simulink model "Copy_of_minimal_rcu_full"  (R2014b)
settings: Solver=ode4  SolverMode=SingleTasking  StartTime=0.0  StopTime=t_sim  FixedStep=sample_time_model  RelTol=1e-3
PreLoadFcn:
  | initModell
InitFcn:
  | initModell
undefined symbols (not defined in the file): FILTER_TAU_EXT, FIXED_FILTER_BANDWIDTH, FIXED_FILTER_BANDWIDTH_OBSERVER, iter, K_INV, KI2TAU_VEC, KS_trq, KT_trq, load_inertia, load_mass, MAX_CURRENT, MIN_SING_VALUE_M_CART, q0, rCEE_i, sample_time_model, sample_time_robot, tau_max
libraries: simulink x69, robotics x15, beasty_sfcns x7, lwr_dynamics x6, trafo3dLib x4, holgersRobLib x3, dspmtrx3 x1, dspinverses x1
(part 3 of 4)

== system Copy_of_minimal_rcu_full/Roboter+controller/controller/Cartesian Impedance Control/Subsystem/Cartesian Compliance Control/Iterative Computation of the 'Stiffness' and Gravity Compensation ==
  note: Notice that q_bar is chosen after the delay block
      | while the tau_qbar is computed before the delay.
      | Therefore, the signals q_bar and tau_qbar fit together
      | and the last iteration step is used only to compute the
      | output not for an update of q_bar!
  q_m : Inport
  type : Inport  Port=2
  niter : Inport  Port=3
  Kd : Inport  Port=4
  Hsd : Inport  Port=5
  load : Inport  Port=6
  tcp_offset : Inport  Port=7
  base_acceleration : Inport  Port=8
  relaxing : Inport  Port=9
  For Iterator : ForIterator  ResetStates=reset  IterationSource=external  IterationLimit=iter+1  ShowIterationPort=off
  Iteration Step : Subsystem
  Iteration for Nolcos Controller : Subsystem
  Terminator : Terminator
  Unit Delay External IC : simulink/Additional Math & Discrete/Additional Discrete/Unit Delay External IC  tsamp=-1
  q_bar : Outport
  tau_qbar : Outport  Port=2
  Jx_bar : Outport  Port=3
  F : Outport  Port=4
  tau_stiffness : Outport  Port=5
  tau_grav : Outport  Port=6
  wires:
  Iteration for Nolcos Controller/3(grav) -> tau_grav/1
  Iteration for Nolcos Controller/6(tau_stiffness) -> tau_stiffness/1
  base_acceleration/1 -> Iteration for Nolcos Controller/7(base_acceleration)
  niter/1 -> For Iterator/1
  Iteration for Nolcos Controller/2(Jx(q)) -> Jx_bar/1
  load/1 -> Iteration for Nolcos Controller/3(load)
  Hsd/1 -> Iteration for Nolcos Controller/2(Hsd)
  Kd/1 -> Iteration for Nolcos Controller/4(Kd)
  Iteration for Nolcos Controller/1(l(q)) -> tau_qbar/1, Iteration Step/1(l(q))
  q_m/1 -> Iteration Step/2(theta), Unit Delay External IC/2
  Unit Delay External IC/1 -> q_bar/1, Iteration for Nolcos Controller/1(q)
  Iteration Step/1(q_bar) -> Unit Delay External IC/1
  type/1 -> Iteration for Nolcos Controller/5(type)
  Iteration for Nolcos Controller/5(F) -> F/1
  tcp_offset/1 -> Iteration for Nolcos Controller/6(tcp_offset)
  relaxing/1 -> Iteration for Nolcos Controller/8(relaxing)
  Iteration for Nolcos Controller/4(Fkin) -> Terminator/1

== system Copy_of_minimal_rcu_full/Roboter+controller/controller/Cartesian Impedance Control/Subsystem/Cartesian Compliance Control/Nullspace Stiffness1 ==
  P_inv : Inport
  0_JT_4 : Inport  Port=2
  dtheta : Inport  Port=3
  M : Inport  Port=4
  desiredVec : Inport  Port=5
  K : Inport  Port=6
  D : Inport  Port=7
  O_T_4 : Inport  Port=8
  W_T_O : Inport  Port=9
  Enable : EnablePort
  Product : Product  Multiplication=Matrix(*)  RndMeth=Zero
  Product2 : Product  Multiplication=Matrix(*)  RndMeth=Zero
  Product4 : Product  Multiplication=Matrix(*)  RndMeth=Zero
  Reshape : Reshape  OutputDimensionality=Column vector (2-D)
  Reshape1 : Reshape  OutputDimensions=[7,6]
  Reshape2 : Reshape  OutputDimensionality=Customize  OutputDimensions=[4,4]
  Reshape3 : Reshape  OutputDimensionality=Column vector (2-D)
  Reshape4 : Reshape
  Reshape5 : Reshape  OutputDimensionality=Customize  OutputDimensions=[7,6]
  Selector : Selector  NumberOfDimensions=2  InputPortWidth=3  IndexOptions=Index vector (dialog),Index vector (dialog)  Indices=[1 2 3],[1 2 3]  OutputSizes=1,1
  Stiffness Calculation : Subsystem
  Transpose : Math  Operator=transpose  SaturateOnIntegerOverflow=on
  tau : Outport  OutDataTypeStr=double  PortDimensions=7  OutputWhenDisabled=reset  InitialOutput=zeros(1,7)
  wires:
  Stiffness Calculation/1(0_F_stiff) -> Product4/2
  M/1 -> Stiffness Calculation/7(Mass)
  K/1 -> Stiffness Calculation/4(Stiffness)
  D/1 -> Stiffness Calculation/6(damping)
  O_T_4/1 -> Stiffness Calculation/2(0_T_4)
  dtheta/1 -> Stiffness Calculation/5(qd)
  Reshape1/1 -> Reshape3/1
  P_inv/1 -> Product2/1
  Product4/1 -> Reshape1/1
  Product2/1 -> Reshape4/1
  0_JT_4/1 -> Reshape5/1
  W_T_O/1 -> Reshape2/1
  Reshape2/1 -> Selector/1
  Product/1 -> Stiffness Calculation/3(Ellbow_Field)
  Selector/1 -> Transpose/1  "W_R_O"
  desiredVec/1 -> Reshape/1
  Transpose/1 -> Product/1  "O_R_W"
  Reshape/1 -> Product/2
  Reshape3/1 -> Product2/2
  Reshape4/1 -> tau/1
  Reshape5/1 -> Stiffness Calculation/1(O_JT_4), Product4/1

== system Copy_of_minimal_rcu_full/Roboter+controller/controller/Cartesian Impedance Control/Subsystem/Cartesian Compliance Control/Singularity Avoidance ==
  qm : Inport
  dqm : Inport  Port=2
  dist : Inport  Port=3
  gain : Inport  Port=4
  d_sing : Inport  Port=5
  Enable : EnablePort  StatesWhenEnabling=reset
  Add : Sum
  Gain : Gain  Gain=-1
  Product : Product  Multiplication=Matrix(*)  RndMeth=Zero
  Product1 : Product  RndMeth=Zero
  Proj. : MATLAB Function  TreatAsAtomicUnit=on
  Reshape : Reshape  OutputDimensionality=Column vector (2-D)
  Reshape1 : Reshape
  Singularity Avoidance : S-Function  FunctionName=lbr_singul_avoid_sfun  Parameters=robot  EnableBusSupport=off  mask{robot=KUKA-LBR}
      mask help: Singularity Avoidance Torques for the DLR lightweight robots
      mask TypeOptions robot: LBR-II | LBR-M | KUKA-LBR
      mask Display:
      | port_label('input', 1, 'q')
      | port_label('input', 2, 'distance')
      | port_label('input', 3, 'gain')
      | port_label('output', 1, 'tau')
      | port_label('output', 2, 'index')
  tau : Outport  OutDataTypeStr=double  PortDimensions=7  OutputWhenDisabled=reset  InitialOutput=zeros(1,7)
  index : Outport  Port=2  OutDataTypeStr=double  PortDimensions=1  OutputWhenDisabled=reset  InitialOutput=0
  wires:
  Singularity Avoidance/1 -> Proj./1(tau), Add/2
  qm/1 -> Singularity Avoidance/1
  dist/1 -> Singularity Avoidance/2
  gain/1 -> Singularity Avoidance/3
  Singularity Avoidance/2 -> index/1
  Proj./1(P) -> Product/1
  dqm/1 -> Reshape/1
  Product/1 -> Reshape1/1
  d_sing/1 -> Product1/1
  Product1/1 -> Gain/1
  Gain/1 -> Add/1
  Add/1 -> tau/1
  Reshape/1 -> Product/2
  Reshape1/1 -> Product1/2

== system Copy_of_minimal_rcu_full/Roboter+controller/controller/Cartesian Impedance Control/Subsystem/Cartesian Compliance Control/cmd ==
  all : Inport
  Embedded MATLAB Function1 : MATLAB Function  TreatAsAtomicUnit=on
  Select K_diag : Selector  InputPortWidth=23  Indices=[3:8]
  Select Type : Selector  InputPortWidth=23
  Select niter : Selector  InputPortWidth=23  Indices=2
  type : Outport
  niter : Outport  Port=2
  K_diag : Outport  Port=3
  wires:
  all/1 -> Select Type/1, Select niter/1, Select K_diag/1
  Select Type/1 -> type/1
  Select niter/1 -> niter/1
  Select K_diag/1 -> Embedded MATLAB Function1/1(K_diag)
  Embedded MATLAB Function1/1(K) -> K_diag/1

== system Copy_of_minimal_rcu_full/Roboter+controller/controller/Cartesian Impedance Control/Subsystem/Cartesian Compliance Control/cmd2 ==
  all : Inport
  Embedded MATLAB Function1 : MATLAB Function  TreatAsAtomicUnit=on
  Select K_diag : Selector  InputPortWidth=23  Indices=[3:8]
  Select Type : Selector  InputPortWidth=23  Indices=23
  Select niter : Selector  InputPortWidth=23  Indices=[9:14]
  xi_diag : Outport
  damping_type : Outport  Port=2
  K_diag : Outport  Port=3
  K_sqrt : Outport  Port=4
  wires:
  Select K_diag/1 -> Embedded MATLAB Function1/1(K_diag)
  Select Type/1 -> damping_type/1
  all/1 -> Select K_diag/1, Select niter/1, Select Type/1
  Embedded MATLAB Function1/1(K) -> K_diag/1
  Embedded MATLAB Function1/2(K_sqrt) -> K_sqrt/1
  Select niter/1 -> xi_diag/1

== system Copy_of_minimal_rcu_full/Roboter+controller/controller/Cartesian Impedance Control/Subsystem/Cartesian Compliance Control/cmd3 ==
  all : Inport
  Select K_diag : Selector  InputPortWidth=23  Indices=16
  Select Type : Selector  InputPortWidth=23  Indices=[17:19]
  Select niter : Selector  InputPortWidth=23  Indices=15
  desiredVec : Outport
  K_NS : Outport  Port=2
  Xi_NS : Outport  Port=3
  wires:
  all/1 -> Select Type/1, Select niter/1, Select K_diag/1
  Select Type/1 -> desiredVec/1
  Select niter/1 -> K_NS/1
  Select K_diag/1 -> Xi_NS/1

== system Copy_of_minimal_rcu_full/Roboter+controller/controller/Cartesian Impedance Control/Subsystem/Cartesian Compliance Control/cmd4 ==
  all : Inport
  Select K_diag : Selector  InputPortWidth=23  Indices=22
  Select Type : Selector  InputPortWidth=23  Indices=20
  Select niter : Selector  InputPortWidth=23  Indices=21
  sing_dist : Outport
  sing_gain : Outport  Port=2
  sing_damp : Outport  Port=3
  wires:
  Select K_diag/1 -> sing_damp/1
  Select niter/1 -> sing_gain/1
  Select Type/1 -> sing_dist/1
  all/1 -> Select K_diag/1, Select niter/1, Select Type/1

== system Copy_of_minimal_rcu_full/Roboter+controller/controller/Cartesian Impedance Control/calculate Feedforward/Numerische Differentiation/Rotate_wrench1 ==
  A_T_B : Inport
  0 : Constant  Value=zeros(3,3)  VectorParams1D=off
  Matrix Concatenation : Concatenate  Mode=Multidimensional array  ConcatenateDimension=2
  Matrix Concatenation1 : Concatenate  Mode=Multidimensional array
  Matrix Concatenation2 : Concatenate  Mode=Multidimensional array  ConcatenateDimension=2
  R : Selector  NumberOfDimensions=2  InputPortWidth=3  IndexOptions=Index vector (dialog),Index vector (dialog)  Indices=[1,2,3],[1 2 3]
  A_R_B : Outport
  wires:
  Matrix Concatenation1/1 -> A_R_B/1
  Matrix Concatenation2/1 -> Matrix Concatenation1/2
  Matrix Concatenation/1 -> Matrix Concatenation1/1
  0/1 -> Matrix Concatenation2/1, Matrix Concatenation/2
  A_T_B/1 -> R/1
  R/1 -> Matrix Concatenation/1, Matrix Concatenation2/2

== system Copy_of_minimal_rcu_full/Roboter+controller/controller/Cartesian Impedance Control/calculate Feedforward/Numerische Differentiation/nan_chk4 ==
  in : Inport
  Add : Sum
  Compare To Zero : simulink/Logic and Bit Operations/Compare To Zero  relop===  OutDataTypeStr=uint8  ZeroCross=off
  Compare To Zero1 : simulink/Logic and Bit Operations/Compare To Zero  relop=>  OutDataTypeStr=uint8  ZeroCross=off
  Constant2 : Constant  Value=sample_time_model
  Discrete Derivative2 : simulink/Discrete/Discrete Derivative  gainval=1.0  ICPrevScaledInput=0.0  InputProcessing=Inherited  OutMin=[]  OutMax=[]  OutDataType=sfix(16)  OutScaling=2^-10  DoSatur=off
  NAN_chk_theta : Display
  Product1 : Product  RndMeth=Zero
  Relational Operator : RelationalOperator  Operator===  OutDataTypeStr=boolean
  Sum of Elements : Sum  Inputs=+
  Switch : Switch  Criteria=u2 > Threshold
  Unit Delay1 : UnitDelay  SampleTime=-1
  in_checked : Outport
  wires:
  Unit Delay1/1 -> Switch/1
  Add/1 -> Unit Delay1/1
  Product1/1 -> Add/2
  Discrete Derivative2/1 -> Product1/1
  Constant2/1 -> Product1/2
  Switch/1 -> Add/1, Discrete Derivative2/1, in_checked/1
  in/1 -> Switch/3, Relational Operator/2, Relational Operator/1
  Relational Operator/1 -> Compare To Zero/1
  Compare To Zero/1 -> Sum of Elements/1
  Sum of Elements/1 -> Compare To Zero1/1
  Compare To Zero1/1 -> Switch/2, NAN_chk_theta/1

== system Copy_of_minimal_rcu_full/Roboter+controller/controller/Cartesian Impedance Control/calculate Feedforward/Numerische Differentiation/numerical differentiation ==
  note: 0_dx = [0_dx_trans; 0_dx_rot]
  note: 0_dx_trans calcualated by numerical differentiation of the position of T_desired
  note: 0_dx_rot calculated by numerical differentiation
      | omegatilde = dR/dt*R^T
  T_des : Inport
  Derivative1 : Derivative
  Derivative2 : Derivative
  Math Function : Math  Operator=transpose  SaturateOnIntegerOverflow=on
  Mux : Mux
  Product3 : Product  Multiplication=Matrix(*)  RndMeth=Zero
  Reshape7 : Reshape  OutputDimensionality=Column vector (2-D)  OutputDimensions=[7,6]
  select_-omega_x : Selector  NumberOfDimensions=2  InputPortWidth=3  IndexOptions=Index vector (dialog),Index vector (dialog)  Indices=3,2  OutputSizes=1,1
  select_omega_y : Selector  NumberOfDimensions=2  InputPortWidth=3  IndexOptions=Index vector (dialog),Index vector (dialog)  Indices=1,3  OutputSizes=1,1
  select_omega_z : Selector  NumberOfDimensions=2  InputPortWidth=3  IndexOptions=Index vector (dialog),Index vector (dialog)  Indices=2,1  OutputSizes=1,1
  select_rot : Selector  NumberOfDimensions=2  InputPortWidth=3  IndexOptions=Index vector (dialog),Index vector (dialog)  Indices=[1:3],[1:3]  OutputSizes=1,1
  select_trans : Selector  NumberOfDimensions=2  InputPortWidth=3  IndexOptions=Index vector (dialog),Index vector (dialog)  Indices=[1:3],4  OutputSizes=1,1
  0_dx : Outport
  wires:
  select_rot/1 -> Derivative1/1, Math Function/1
  Derivative1/1 -> Product3/1
  Math Function/1 -> Product3/2
  select_trans/1 -> Derivative2/1
  Product3/1 -> select_-omega_x/1, select_omega_y/1, select_omega_z/1
  select_-omega_x/1 -> Mux/2
  select_omega_z/1 -> Mux/4
  select_omega_y/1 -> Mux/3
  Derivative2/1 -> Mux/1  "0_dx_trans"
  Mux/1 -> Reshape7/1
  T_des/1 -> select_rot/1, select_trans/1
  Reshape7/1 -> 0_dx/1

== system Copy_of_minimal_rcu_full/Roboter+controller/controller/Cartesian Impedance Control/easy interpolate/easy interpolator inside/correct sign ==
  In1 : Inport
  In2 : Inport  Port=2
  Constant2 : Constant
  Constant3 : Constant  Value=-1
  Relational Operator : RelationalOperator  Operator=<  OutDataTypeStr=boolean
  Switch : Switch  Criteria=u2 > Threshold
  Out1 : Outport
  wires:
  Switch/1 -> Out1/1
  In1/1 -> Relational Operator/1
  Constant2/1 -> Switch/1
  Relational Operator/1 -> Switch/2
  Constant3/1 -> Switch/3
  In2/1 -> Relational Operator/2

== system Copy_of_minimal_rcu_full/Roboter+controller/controller/Cartesian Impedance Control/easy interpolate/easy interpolator inside/memorize last ==
  In1 : Inport
  Detect Change : simulink/Logic and Bit Operations/Detect Change  vinit=0  InputProcessing=Inherited  OutDataTypeStr=uint8
  Display1 : Display
  Display2 : Display
  Display3 : Display
  Scope : Scope
      settings: YMin=1  YMax=1
  Triggered Subsystem : Subsystem  TreatAsAtomicUnit=on
  Unit Delay : UnitDelay  SampleTime=-1
  Out1 : Outport
  wires:
  In1/1 -> Display3/1, Detect Change/1, Unit Delay/1
  Detect Change/1 -> Triggered Subsystem/Trigger, Display1/1, Scope/1
  Unit Delay/1 -> Triggered Subsystem/1(In1)
  Triggered Subsystem/1(Out1) -> Out1/1, Display2/1

== system Copy_of_minimal_rcu_full/Roboter+controller/controller/Joint Impedance/JOINT_IMPEDANCE_CONTROL/Joint Compliance Control/Damping Design via Generalized Eigenvalues ==
  note: The following is satisfied:
      |   V'BV=I
      |   inv(V)*inv(B)*A*V=diag(lam)
      |   H=inv(V')=B*V-->B=H*H' and B=inv(V')*inv(V)
      |   The damping should thus be chosen as Dc = H*diag(d0)*H'
  M : Inport
  K : Inport  Port=2
  damp_fac : Inport  Port=3
  Damping Design via Generalized Eigenvalues QR right : Subsystem
  D : Outport
  wires:
  damp_fac/1 -> Damping Design via Generalized Eigenvalues QR right/3(damp_fac)
  K/1 -> Damping Design via Generalized Eigenvalues QR right/1(K)
  M/1 -> Damping Design via Generalized Eigenvalues QR right/2(M)
  Damping Design via Generalized Eigenvalues QR right/1(D) -> D/1

== system Copy_of_minimal_rcu_full/Roboter+controller/controller/Joint Impedance/JOINT_IMPEDANCE_CONTROL/Joint Compliance Control/NAN_checks ==
  D : Inport
  qm : Inport  Port=2
  dqm : Inport  Port=3
  qm_d : Inport  Port=4
  K_diag : Inport  Port=5
  stiffness correction : Inport  Port=6
  g(theta) : Inport  Port=7
  tau : Inport  Port=8
  NAN_chk_K_diag : Display
  NAN_chk_damping : Display
  NAN_chk_gravitation : Display
  NAN_chk_stiffness correction : Display
  NAN_chk_tau_joint_impedance : Display
  NAN_chk_theta_dot_measured : Display
  NAN_chk_theta_measured : Display
  NAN_chk_theta_measured_desired : Display
  hold_zero_if_nan_or_inf1 : Subsystem
  hold_zero_if_nan_or_inf2 : Subsystem
  hold_zero_if_nan_or_inf3 : Subsystem
  hold_zero_if_nan_or_inf4 : Subsystem
  hold_zero_if_nan_or_inf5 : Subsystem
  hold_zero_if_nan_or_inf6 : Subsystem
  hold_zero_if_nan_or_inf7 : Subsystem
  hold_zero_if_nan_or_inf8 : Subsystem
  wires:
  hold_zero_if_nan_or_inf2/1(Out1) -> NAN_chk_theta_measured/1
  hold_zero_if_nan_or_inf3/1(Out1) -> NAN_chk_theta_dot_measured/1
  hold_zero_if_nan_or_inf4/1(Out1) -> NAN_chk_theta_measured_desired/1
  hold_zero_if_nan_or_inf5/1(Out1) -> NAN_chk_K_diag/1
  hold_zero_if_nan_or_inf6/1(Out1) -> NAN_chk_damping/1
  hold_zero_if_nan_or_inf7/1(Out1) -> NAN_chk_stiffness correction/1
  hold_zero_if_nan_or_inf8/1(Out1) -> NAN_chk_gravitation/1
  qm/1 -> hold_zero_if_nan_or_inf2/1(In1)
  dqm/1 -> hold_zero_if_nan_or_inf3/1(In1)
  qm_d/1 -> hold_zero_if_nan_or_inf4/1(In1)
  K_diag/1 -> hold_zero_if_nan_or_inf5/1(In1)
  D/1 -> hold_zero_if_nan_or_inf6/1(In1)
  stiffness correction/1 -> hold_zero_if_nan_or_inf7/1(In1)
  g(theta)/1 -> hold_zero_if_nan_or_inf8/1(In1)
  hold_zero_if_nan_or_inf1/1(Out1) -> NAN_chk_tau_joint_impedance/1
  tau/1 -> hold_zero_if_nan_or_inf1/1(In1)

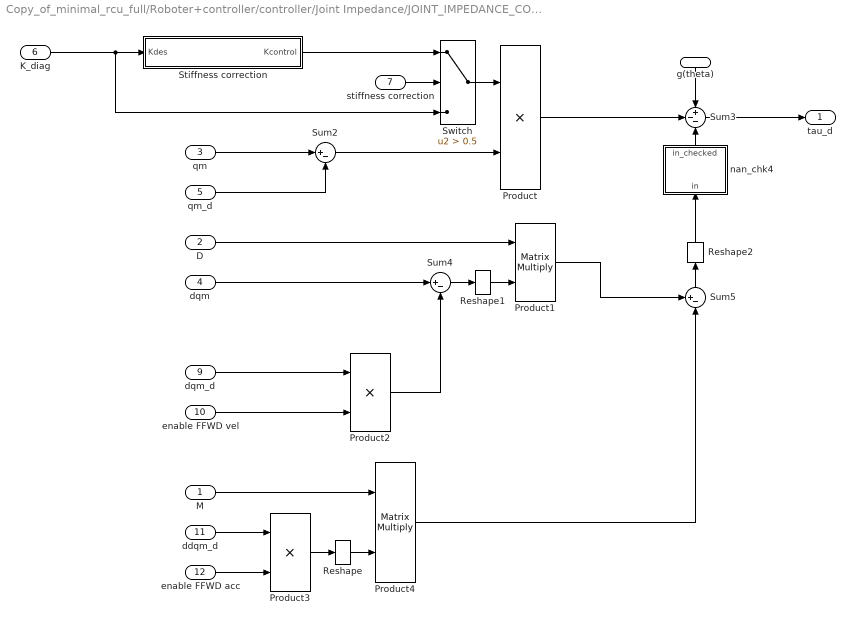
== system Copy_of_minimal_rcu_full/Roboter+controller/controller/Joint Impedance/JOINT_IMPEDANCE_CONTROL/Joint Compliance Control/Pragmatic Solution ==
  M : Inport
  D : Inport  Port=2
  qm : Inport  Port=3
  dqm : Inport  Port=4
  qm_d : Inport  Port=5
  K_diag : Inport  Port=6
  stiffness correction : Inport  Port=7
  g(theta) : Inport  Port=8
  dqm_d : Inport  Port=9
  enable FFWD vel : Inport  Port=10
  ddqm_d : Inport  Port=11
  enable FFWD acc : Inport  Port=12
  Product : Product  RndMeth=Zero
  Product1 : Product  Multiplication=Matrix(*)  RndMeth=Zero
  Product2 : Product  RndMeth=Zero
  Product3 : Product  RndMeth=Zero
  Product4 : Product  Multiplication=Matrix(*)  RndMeth=Zero
  Reshape : Reshape  OutputDimensionality=Column vector (2-D)
  Reshape1 : Reshape  OutputDimensionality=Column vector (2-D)
  Reshape2 : Reshape
  Stiffness correction : MATLAB Function  TreatAsAtomicUnit=on
  Sum2 : Sum  Inputs=|+-
  Sum3 : Sum  Inputs=+--
  Sum4 : Sum  Inputs=|+-
  Sum5 : Sum  Inputs=+-|
  Switch : Switch  Criteria=u2 > Threshold  Threshold=0.5
  nan_chk4 : Subsystem
  tau_d : Outport
  wires:
  Sum2/1 -> Product/2
  Sum3/1 -> tau_d/1
  qm/1 -> Sum2/1
  qm_d/1 -> Sum2/2
  D/1 -> Product1/1
  K_diag/1 -> Stiffness correction/1(Kdes), Switch/3
  stiffness correction/1 -> Switch/2
  Stiffness correction/1(Kcontrol) -> Switch/1
  Switch/1 -> Product/1
  Sum4/1 -> Reshape1/1
  dqm/1 -> Sum4/1
  dqm_d/1 -> Product2/1
  enable FFWD vel/1 -> Product2/2
  Product2/1 -> Sum4/2
  ddqm_d/1 -> Product3/1
  enable FFWD acc/1 -> Product3/2
  M/1 -> Product4/1
  Product3/1 -> Reshape/1
  Sum5/1 -> Reshape2/1
  Product1/1 -> Sum5/1
  Product4/1 -> Sum5/2
  Product/1 -> Sum3/2
  nan_chk4/1(in_checked) -> Sum3/3
  g(theta)/1 -> Sum3/1
  Reshape/1 -> Product4/2
  Reshape1/1 -> Product1/2
  Reshape2/1 -> nan_chk4/1(in)

== system Copy_of_minimal_rcu_full/Roboter+controller/controller/Joint Impedance/JOINT_IMPEDANCE_CONTROL/Joint Compliance Control/cmd ==
  all : Inport
  Demux : Demux  Outputs=5
  Signal Specification1 : SignalSpecification  Dimensions=7
  Signal Specification{2..5} (4 alike) : SignalSpecification  Dimensions=1
  niter : Terminator
  K_diag : Outport
  xi_diag : Outport  Port=2
  delay : Outport  Port=3
  stiffness_correction : Outport  Port=4
  wires:
  Signal Specification1/1 -> K_diag/1
  all/1 -> Demux/1
  Signal Specification2/1 -> xi_diag/1
  Signal Specification3/1 -> niter/1
  Signal Specification4/1 -> stiffness_correction/1
  Signal Specification5/1 -> delay/1
  Demux/1 -> Signal Specification1/1
  Demux/2 -> Signal Specification2/1
  Demux/3 -> Signal Specification3/1
  Demux/4 -> Signal Specification4/1
  Demux/5 -> Signal Specification5/1

== system Copy_of_minimal_rcu_full/Roboter+controller/controller/Joint Impedance/Velocity Filter/Subsystem/Weighted Sample Time Math ==

== system Copy_of_minimal_rcu_full/Roboter+controller/robot_simulation/Dynamics/ZUSTANDSREGLER1/controller cart impedance/num. derivative ==
  x[n] : Inport
  CG_0 : Inport  Port=2
  reset : Inport  Port=3
  Sum5 : Sum  Inputs=+-  SaturateOnIntegerOverflow=on  InputSameDT=on  OutDataTypeStr=Inherit: Same as first input
  Unit Delay Resettable External IC : simulink/Additional Math & Discrete/Additional Discrete/Unit Delay Resettable External IC  tsamp=-1
  x_coeff : Gain  Gain=1/h  SaturateOnIntegerOverflow=on  OutDataTypeStr=Inherit: Same as input  ParamDataTypeStr=Inherit: Same as input
  x_coeff1 : Gain  Gain=1/h  SaturateOnIntegerOverflow=on  OutDataTypeStr=Inherit: Same as input  ParamDataTypeStr=Inherit: Same as input
  y[n] : Outport  InitialOutput=0
  wires:
  Unit Delay Resettable External IC/1 -> Sum5/2  "y[n-1]"
  x[n]/1 -> x_coeff/1
  Sum5/1 -> y[n]/1
  x_coeff/1 -> Sum5/1, Unit Delay Resettable External IC/1
  CG_0/1 -> x_coeff1/1
  x_coeff1/1 -> Unit Delay Resettable External IC/3
  reset/1 -> Unit Delay Resettable External IC/2

== system Copy_of_minimal_rcu_full/Roboter+controller/robot_simulation/Dynamics/ZUSTANDSREGLER1/controller cart impedance/num. derivative2 ==
  x[n] : Inport
  CG_0 : Inport  Port=2
  reset : Inport  Port=3
  Sum5 : Sum  Inputs=+-  SaturateOnIntegerOverflow=on  InputSameDT=on  OutDataTypeStr=Inherit: Same as first input
  Unit Delay Resettable External IC : simulink/Additional Math & Discrete/Additional Discrete/Unit Delay Resettable External IC  tsamp=-1
  x_coeff : Gain  Gain=1/h  SaturateOnIntegerOverflow=on  OutDataTypeStr=Inherit: Same as input  ParamDataTypeStr=Inherit: Same as input
  x_coeff1 : Gain  Gain=1/h  SaturateOnIntegerOverflow=on  OutDataTypeStr=Inherit: Same as input  ParamDataTypeStr=Inherit: Same as input
  y[n] : Outport  InitialOutput=0
  wires:
  x_coeff/1 -> Sum5/1, Unit Delay Resettable External IC/1
  Sum5/1 -> y[n]/1
  x[n]/1 -> x_coeff/1
  Unit Delay Resettable External IC/1 -> Sum5/2  "y[n-1]"
  CG_0/1 -> x_coeff1/1
  x_coeff1/1 -> Unit Delay Resettable External IC/3
  reset/1 -> Unit Delay Resettable External IC/2

== system Copy_of_minimal_rcu_full/Roboter+controller/controller/Cartesian Impedance Control/Subsystem/Cartesian Compliance Control/Cartesian Damping/Cartesian mass matrix ==
  Jacobian : Inport
  Mass : Inport  Port=2
  Divide : Product  Inputs=/  Multiplication=Matrix(*)
  Math Function : Math  Operator=transpose  SaturateOnIntegerOverflow=on
  Product1 : Product  Multiplication=Matrix(*)  RndMeth=Zero
  Product2 : Product  Multiplication=Matrix(*)  RndMeth=Zero
  Rate Transition5 : RateTransition
  Rate Transition6 : RateTransition  OutPortSampleTime=sample_time_model
  Rate Transition7 : RateTransition  OutPortSampleTime=sample_time_model
  Rate Transition8 : RateTransition  OutPortSampleTime=sample_time_model
  Subsystem1 : Subsystem
  not_singular : Outport
  Mass_cart : Outport  Port=2
  Mass_cart_sqrt : Outport  Port=3
  wires:
  Divide/1 -> Product2/2
  Math Function/1 -> Product1/2
  Product2/1 -> Product1/1
  Product1/1 -> Rate Transition5/1
  Subsystem1/1(not_singular) -> Rate Transition6/1
  Subsystem1/2(inv_matrix) -> Rate Transition7/1
  Subsystem1/3(inv_matrix_sqrt) -> Rate Transition8/1
  Mass/1 -> Divide/1
  Jacobian/1 -> Product2/1, Math Function/1
  Rate Transition5/1 -> Subsystem1/1(in_matrix)
  Rate Transition6/1 -> not_singular/1
  Rate Transition7/1 -> Mass_cart/1
  Rate Transition8/1 -> Mass_cart_sqrt/1

== system Copy_of_minimal_rcu_full/Roboter+controller/controller/Cartesian Impedance Control/Subsystem/Cartesian Compliance Control/Cartesian Damping/Damping Design via Generalized Eigenvalues ==
  note: The following is satisfied:
      |   V'BV=I
      |   inv(V)*inv(B)*A*V=diag(lam)
      |   H=inv(V')=B*V-->B=H*H' and B=inv(V')*inv(V)
      |   The damping should thus be chosen as Dc = H*diag(d0)*H'
  K : Inport
  M : Inport  Port=2
  damp_fac : Inport  Port=3
  Enable : EnablePort  StatesWhenEnabling=reset
  Damping Design via Generalized Eigenvalues QR right : Subsystem
  D : Outport
  wires:
  Damping Design via Generalized Eigenvalues QR right/1(D) -> D/1
  M/1 -> Damping Design via Generalized Eigenvalues QR right/2(M)
  K/1 -> Damping Design via Generalized Eigenvalues QR right/1(K)
  damp_fac/1 -> Damping Design via Generalized Eigenvalues QR right/3(damp_fac)

== system Copy_of_minimal_rcu_full/Roboter+controller/controller/Cartesian Impedance Control/Subsystem/Cartesian Compliance Control/Cartesian Damping/Damping_design ==
  Mass_sqrt : Inport
  K_X_sqrt : Inport  Port=2
  D_xi : Inport  Port=3
  Enable : EnablePort  StatesWhenEnabling=reset
  Add1 : Sum
  Embedded MATLAB Function1 : MATLAB Function  TreatAsAtomicUnit=on
  Product{1..4} (4 alike) : Product  Multiplication=Matrix(*)  RndMeth=Zero
  D_X : Outport
  wires:
  Mass_sqrt/1 -> Product4/2, Product1/1
  Product1/1 -> Add1/1
  Product2/1 -> Add1/2
  Add1/1 -> D_X/1
  Product4/1 -> Product2/2
  Product3/1 -> Product1/2
  D_xi/1 -> Embedded MATLAB Function1/1(u)
  K_X_sqrt/1 -> Product2/1, Product3/2
  Embedded MATLAB Function1/1(y) -> Product4/1, Product3/1

== system Copy_of_minimal_rcu_full/Roboter+controller/controller/Cartesian Impedance Control/Subsystem/Cartesian Compliance Control/Iterative Computation of the 'Stiffness' and Gravity Compensation/Iteration Step ==
  l(q) : Inport
  theta : Inport  Port=2
  Gain : Gain  Gain=K_INV
  Sum : Sum  Inputs=|+-
  q_bar : Outport
  wires:
  Gain/1 -> Sum/2
  l(q)/1 -> Gain/1
  Sum/1 -> q_bar/1
  theta/1 -> Sum/1

== system Copy_of_minimal_rcu_full/Roboter+controller/controller/Cartesian Impedance Control/Subsystem/Cartesian Compliance Control/Iterative Computation of the 'Stiffness' and Gravity Compensation/Iteration for Nolcos Controller ==
  q : Inport
  Hsd : Inport  Port=2
  load : Inport  Port=3
  Kd : Inport  Port=4
  type : Inport  Port=5
  tcp_offset : Inport  Port=6
  base_acceleration : Inport  Port=7
  relaxing : Inport  Port=8
  Compare To Constant : simulink/Logic and Bit Operations/Compare To Constant  relop===  const=1  OutDataTypeStr=uint8  ZeroCross=off
  Compare To Constant1 : simulink/Logic and Bit Operations/Compare To Constant  relop===  const=2  OutDataTypeStr=uint8  ZeroCross=off
  Euler Angle Stiffness : Subsystem  TreatAsAtomicUnit=on
  LBR M Components2 : Subsystem
  Multiport Switch : MultiPortSwitch  Inputs=2
  Multiport Switch1 : MultiPortSwitch  Inputs=2
  Multiport Switch2 : MultiPortSwitch  Inputs=2
  Saturation : Saturate  UpperLimit=2  LowerLimit=1
  Spatial Stiffness : Subsystem  TreatAsAtomicUnit=on
  Sum3 : Sum  Inputs=++|
  Terminator : Terminator
  l(q) : Outport
  Jx(q) : Outport  Port=2
  grav : Outport  Port=3
  Fkin : Outport  Port=4
  F : Outport  Port=5
  tau_stiffness : Outport  Port=6
  wires:
  base_acceleration/1 -> LBR M Components2/4(base_acceleration)
  Kd/1 -> Euler Angle Stiffness/4(K), Spatial Stiffness/4(K)
  load/1 -> LBR M Components2/2(load)
  LBR M Components2/3(grav) -> grav/1, Sum3/2  "gravity"
  Sum3/1 -> l(q)/1
  Hsd/1 -> Euler Angle Stiffness/1(Hsd), Spatial Stiffness/1(Hsd)
  LBR M Components2/2(J) -> Euler Angle Stiffness/3(Jbody), Spatial Stiffness/3(Jbody)
  LBR M Components2/1(Fkin) -> Fkin/1, Euler Angle Stiffness/2(Fkin), Spatial Stiffness/2(Fkin)
  q/1 -> LBR M Components2/1(q)
  type/1 -> Saturation/1
  Compare To Constant1/1 -> Spatial Stiffness/Enable
  Compare To Constant/1 -> Euler Angle Stiffness/Enable
  Euler Angle Stiffness/1(tau) -> Multiport Switch/2
  Euler Angle Stiffness/2(J) -> Multiport Switch1/2
  Spatial Stiffness/1(tau) -> Multiport Switch/3
  Spatial Stiffness/2(J) -> Multiport Switch1/3
  Multiport Switch/1 -> tau_stiffness/1, Sum3/1  "stiffness"
  Multiport Switch1/1 -> Jx(q)/1
  Saturation/1 -> Compare To Constant1/1, Multiport Switch/1, Multiport Switch1/1, Multiport Switch2/1, Compare To Constant/1
  Euler Angle Stiffness/4(F) -> Multiport Switch2/2
  Spatial Stiffness/3(F) -> Multiport Switch2/3
  Multiport Switch2/1 -> F/1
  tcp_offset/1 -> LBR M Components2/3(tcp_offset)
  relaxing/1 -> Euler Angle Stiffness/5(relaxing), Spatial Stiffness/5(relaxing)
  Euler Angle Stiffness/3(x) -> Terminator/1

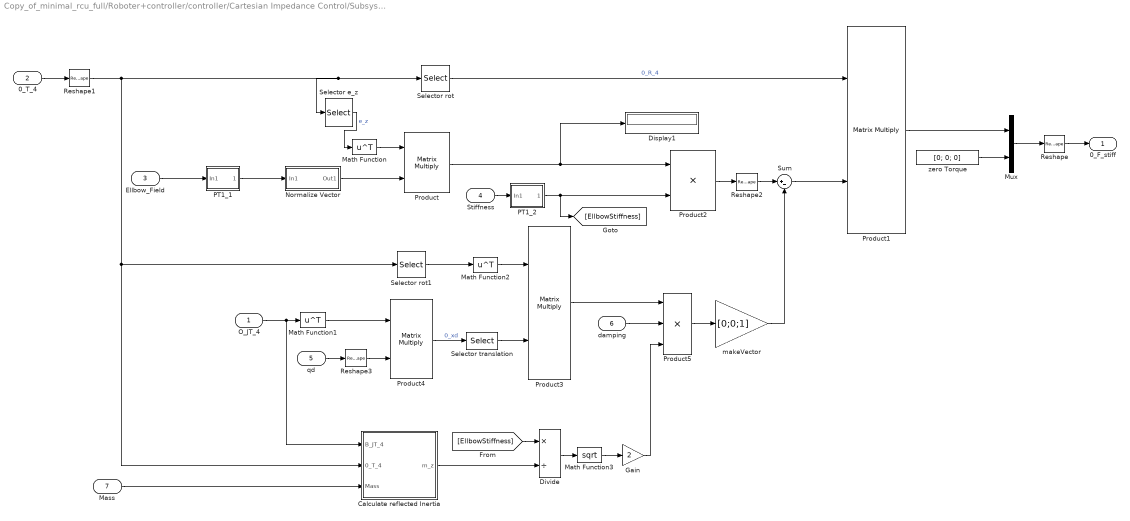
== system Copy_of_minimal_rcu_full/Roboter+controller/controller/Cartesian Impedance Control/Subsystem/Cartesian Compliance Control/Nullspace Stiffness1/Stiffness Calculation ==
  O_JT_4 : Inport
  0_T_4 : Inport  Port=2
  Ellbow_Field : Inport  Port=3
  Stiffness : Inport  Port=4
  qd : Inport  Port=5
  damping : Inport  Port=6
  Mass : Inport  Port=7
  Calculate reflected Inertia : Subsystem
  Display1 : Display
  Divide : Product  Inputs=*/
  Gain : Gain  Gain=2
  Math Function : Math  Operator=transpose  SaturateOnIntegerOverflow=on
  Math Function1 : Math  Operator=transpose  SaturateOnIntegerOverflow=on
  Math Function2 : Math  Operator=transpose  SaturateOnIntegerOverflow=on
  Math Function3 : Math  Operator=sqrt  SaturateOnIntegerOverflow=on
  Mux : Mux  Inputs=2
  Normalize Vector : Subsystem  mask(Normalize Vector){maxzero=0}
      mask prompts: maxzero "Maximum modulus to treat vector as zero:"
      mask help:
      | Normalize a vector.
      | Output is the unit vector parallel to the input vector. Input can be vector of any size.
      | If the modulus of the input is lower or equal than specified, the output is set to zeros(size(u)).
      mask Help: helpview(fullfile(docroot, 'toolbox', 'vr', 'vr.map'), 'vr_normalizevector');
      mask Display: disp('Normalize')
  PT1_1 : Subsystem
  PT1_2 : Subsystem
  Product{,1,3..4} (4 alike) : Product  Multiplication=Matrix(*)  RndMeth=Zero
  Product2 : Product  RndMeth=Zero
  Product5 : Product  Inputs=3  RndMeth=Zero
  Reshape : Reshape  OutputDimensionality=Column vector (2-D)
  Reshape1 : Reshape  OutputDimensionality=Customize  OutputDimensions=[3,4]
  Reshape2 : Reshape  OutputDimensionality=Column vector (2-D)
  Reshape3 : Reshape  OutputDimensionality=Column vector (2-D)
  Selector e_z : Selector  NumberOfDimensions=2  InputPortWidth=3  IndexOptions=Index vector (dialog),Index vector (dialog)  Indices=[1 2 3],3  OutputSizes=1,1
  Selector rot : Selector  NumberOfDimensions=2  InputPortWidth=3  IndexOptions=Index vector (dialog),Index vector (dialog)  Indices=[1 2 3],[1 2 3]  OutputSizes=1,1
  Selector rot1 : Selector  NumberOfDimensions=2  InputPortWidth=3  IndexOptions=Index vector (dialog),Index vector (dialog)  Indices=[1 2 3],[1 2 3]  OutputSizes=1,1
  Selector translation : Selector  InputPortWidth=6  Indices=[1 2 3]
  Sum : Sum  Inputs=|+-
  makeVector : Gain  Gain=[0;0;1]
  zero Torque : Constant  Value=[0; 0; 0]
  0_F_stiff : Outport  OutDataTypeStr=double  PortDimensions=[6 1]
  wires:
  Gain/1 -> Product5/3
  Math Function3/1 -> Gain/1
  Divide/1 -> Math Function3/1
  Calculate reflected Inertia/1(m_z) -> Divide/2
  [EllbowStiffness] -> Divide/1
  Selector rot1/1 -> Math Function2/1
  Mass/1 -> Calculate reflected Inertia/3(Mass)
  makeVector/1 -> Sum/2
  Reshape2/1 -> Sum/1
  Sum/1 -> Product1/2
  Math Function2/1 -> Product3/1
  Product5/1 -> makeVector/1
  Product3/1 -> Product5/1
  Selector translation/1 -> Product3/2
  Product4/1 -> Selector translation/1  "0_xd"
  qd/1 -> Reshape3/1
  O_JT_4/1 -> Calculate reflected Inertia/1(B_JT_4), Math Function1/1
  Math Function1/1 -> Product4/1
  Product/1 -> Product2/1, Display1/1
  Stiffness/1 -> PT1_2/1(In1)
  Product2/1 -> Reshape2/1
  Reshape/1 -> 0_F_stiff/1
  0_T_4/1 -> Reshape1/1
  zero Torque/1 -> Mux/2
  Product1/1 -> Mux/1
  Selector rot/1 -> Product1/1  "0_R_4"
  Math Function/1 -> Product/1
  Mux/1 -> Reshape/1
  Selector e_z/1 -> Math Function/1  "e_z"
  Normalize Vector/1(Out1) -> Product/2
  damping/1 -> Product5/2
  PT1_2/1(Out1) -> [EllbowStiffness], Product2/2
  Reshape1/1 -> Selector rot1/1, Calculate reflected Inertia/2(0_T_4), Selector rot/1, Selector e_z/1
  PT1_1/1(Out1) -> Normalize Vector/1(In1)
  Ellbow_Field/1 -> PT1_1/1(In1)
  Reshape3/1 -> Product4/2

== system Copy_of_minimal_rcu_full/Roboter+controller/controller/Cartesian Impedance Control/easy interpolate/easy interpolator inside/memorize last/Triggered Subsystem ==
  In1 : Inport
  Trigger : TriggerPort
  Out1 : Outport
  wires:
  In1/1 -> Out1/1

== system Copy_of_minimal_rcu_full/Roboter+controller/controller/Joint Impedance/JOINT_IMPEDANCE_CONTROL/Joint Compliance Control/Damping Design via Generalized Eigenvalues/Damping Design via Generalized Eigenvalues QR right ==
  K : Inport
  M : Inport  Port=2
  damp_fac : Inport  Port=3
  2*Damping Fac : Gain  Gain=2
  Embedded MATLAB Function : MATLAB Function  TreatAsAtomicUnit=on
  Math Function1 : Math  Operator=sqrt  OutputSignalType=real  SaturateOnIntegerOverflow=on
  Product1 : Product  Inputs=***  Multiplication=Matrix(*)  RndMeth=Zero
  Product2 : Product  Inputs=**  Multiplication=Matrix(*)  RndMeth=Zero
  Product3 : Product  Inputs=**  RndMeth=Zero
  Rate Transition : RateTransition  OutPortSampleTime=0.001
  Rate Transition1 : RateTransition  OutPortSampleTime=0.001
  Rate Transition2 : RateTransition  OutPortSampleTime=sample_time_model
  Rate Transition3 : RateTransition  OutPortSampleTime=sample_time_model
  Rate Transition4 : RateTransition  OutPortSampleTime=sample_time_model
  Subsystem : Subsystem  SystemSampleTime=0.001
  D : Outport
  wires:
  Subsystem/3(Vinv) -> Rate Transition3/1
  Embedded MATLAB Function/1(y) -> Product1/2  "C"
  Product2/1 -> Product1/1
  damp_fac/1 -> Product3/2
  Product3/1 -> Embedded MATLAB Function/1(u)
  2*Damping Fac/1 -> Product3/1
  Product1/1 -> D/1
  K/1 -> Rate Transition/1
  Subsystem/2(lambda) -> Rate Transition2/1
  Subsystem/1(V) -> Rate Transition4/1
  Math Function1/1 -> 2*Damping Fac/1
  M/1 -> Rate Transition1/1, Product2/1
  Rate Transition/1 -> Subsystem/1(A)
  Rate Transition1/1 -> Subsystem/2(B)
  Rate Transition3/1 -> Product1/3
  Rate Transition2/1 -> Math Function1/1
  Rate Transition4/1 -> Product2/2

== system Copy_of_minimal_rcu_full/Roboter+controller/controller/Joint Impedance/JOINT_IMPEDANCE_CONTROL/Joint Compliance Control/NAN_checks/hold_zero_if_nan_or_inf1 ==
  In1 : Inport
  Compare To Zero6 : simulink/Logic and Bit Operations/Compare To Zero  relop===  OutDataTypeStr=uint8  ZeroCross=off
  Compare To Zero8 : simulink/Logic and Bit Operations/Compare To Zero  relop===  OutDataTypeStr=uint8  ZeroCross=off
  Data Type Conversion1 : DataTypeConversion
  Display5 : Display
  Hold1 : Stateflow chart  TreatAsAtomicUnit=on
  Mux1 : Mux  Inputs=2
  Nan Check : simulink/Model Verification/Check  Static Range  Description=-inf < u < inf  max=inf  max_included=off  min=-inf  min_included=off  enabled=on  stopWhenAssertionFail=off  export=on  icon=graphic
  Sum of Elements : Sum  Inputs=+
  Unit Delay1 : UnitDelay  SampleTime=-1
  reset1 : Constant  Value=0
  Out1 : Outport
  wires:
  In1/1 -> Nan Check/1
  Nan Check/1 -> Display5/1, Compare To Zero6/1
  Compare To Zero6/1 -> Sum of Elements/1
  reset1/1 -> Mux1/2
  Mux1/1 -> Hold1/Trigger
  Hold1/1(error) -> Compare To Zero8/1
  Data Type Conversion1/1 -> Mux1/1
  Unit Delay1/1 -> Data Type Conversion1/1
  Compare To Zero8/1 -> Out1/1
  Sum of Elements/1 -> Unit Delay1/1

== system Copy_of_minimal_rcu_full/Roboter+controller/controller/Joint Impedance/JOINT_IMPEDANCE_CONTROL/Joint Compliance Control/NAN_checks/hold_zero_if_nan_or_inf2 ==
  In1 : Inport
  Compare To Zero6 : simulink/Logic and Bit Operations/Compare To Zero  relop===  OutDataTypeStr=uint8  ZeroCross=off
  Compare To Zero8 : simulink/Logic and Bit Operations/Compare To Zero  relop===  OutDataTypeStr=uint8  ZeroCross=off
  Data Type Conversion1 : DataTypeConversion
  Display5 : Display
  Hold1 : Stateflow chart  TreatAsAtomicUnit=on
  Mux1 : Mux  Inputs=2
  Nan Check : simulink/Model Verification/Check  Static Range  Description=-inf < u < inf  max=inf  max_included=off  min=-inf  min_included=off  enabled=on  stopWhenAssertionFail=off  export=on  icon=graphic
  Sum of Elements : Sum  Inputs=+
  Unit Delay1 : UnitDelay  SampleTime=-1
  reset1 : Constant  Value=0
  Out1 : Outport
  wires:
  Sum of Elements/1 -> Unit Delay1/1
  Compare To Zero8/1 -> Out1/1
  Unit Delay1/1 -> Data Type Conversion1/1
  Data Type Conversion1/1 -> Mux1/1
  Hold1/1(error) -> Compare To Zero8/1
  Mux1/1 -> Hold1/Trigger
  reset1/1 -> Mux1/2
  Compare To Zero6/1 -> Sum of Elements/1
  Nan Check/1 -> Compare To Zero6/1, Display5/1
  In1/1 -> Nan Check/1

== system Copy_of_minimal_rcu_full/Roboter+controller/controller/Joint Impedance/JOINT_IMPEDANCE_CONTROL/Joint Compliance Control/NAN_checks/hold_zero_if_nan_or_inf3 ==
  In1 : Inport
  Compare To Zero6 : simulink/Logic and Bit Operations/Compare To Zero  relop===  OutDataTypeStr=uint8  ZeroCross=off
  Compare To Zero8 : simulink/Logic and Bit Operations/Compare To Zero  relop===  OutDataTypeStr=uint8  ZeroCross=off
  Data Type Conversion1 : DataTypeConversion
  Display5 : Display
  Hold1 : Stateflow chart  TreatAsAtomicUnit=on
  Mux1 : Mux  Inputs=2
  Nan Check : simulink/Model Verification/Check  Static Range  Description=-inf < u < inf  max=inf  max_included=off  min=-inf  min_included=off  enabled=on  stopWhenAssertionFail=off  export=on  icon=graphic
  Sum of Elements : Sum  Inputs=+
  Unit Delay1 : UnitDelay  SampleTime=-1
  reset1 : Constant  Value=0
  Out1 : Outport
  wires:
  In1/1 -> Nan Check/1
  Nan Check/1 -> Display5/1, Compare To Zero6/1
  Compare To Zero6/1 -> Sum of Elements/1
  reset1/1 -> Mux1/2
  Mux1/1 -> Hold1/Trigger
  Hold1/1(error) -> Compare To Zero8/1
  Data Type Conversion1/1 -> Mux1/1
  Unit Delay1/1 -> Data Type Conversion1/1
  Compare To Zero8/1 -> Out1/1
  Sum of Elements/1 -> Unit Delay1/1

== system Copy_of_minimal_rcu_full/Roboter+controller/controller/Joint Impedance/JOINT_IMPEDANCE_CONTROL/Joint Compliance Control/NAN_checks/hold_zero_if_nan_or_inf4 ==
  In1 : Inport
  Compare To Zero6 : simulink/Logic and Bit Operations/Compare To Zero  relop===  OutDataTypeStr=uint8  ZeroCross=off
  Compare To Zero8 : simulink/Logic and Bit Operations/Compare To Zero  relop===  OutDataTypeStr=uint8  ZeroCross=off
  Data Type Conversion1 : DataTypeConversion
  Display5 : Display
  Hold1 : Stateflow chart  TreatAsAtomicUnit=on
  Mux1 : Mux  Inputs=2
  Nan Check : simulink/Model Verification/Check  Static Range  Description=-inf < u < inf  max=inf  max_included=off  min=-inf  min_included=off  enabled=on  stopWhenAssertionFail=off  export=on  icon=graphic
  Sum of Elements : Sum  Inputs=+
  Unit Delay1 : UnitDelay  SampleTime=-1
  reset1 : Constant  Value=0
  Out1 : Outport
  wires:
  Sum of Elements/1 -> Unit Delay1/1
  Compare To Zero8/1 -> Out1/1
  Unit Delay1/1 -> Data Type Conversion1/1
  Data Type Conversion1/1 -> Mux1/1
  Hold1/1(error) -> Compare To Zero8/1
  Mux1/1 -> Hold1/Trigger
  reset1/1 -> Mux1/2
  Compare To Zero6/1 -> Sum of Elements/1
  Nan Check/1 -> Compare To Zero6/1, Display5/1
  In1/1 -> Nan Check/1

== system Copy_of_minimal_rcu_full/Roboter+controller/controller/Joint Impedance/JOINT_IMPEDANCE_CONTROL/Joint Compliance Control/NAN_checks/hold_zero_if_nan_or_inf5 ==
  In1 : Inport
  Compare To Zero6 : simulink/Logic and Bit Operations/Compare To Zero  relop===  OutDataTypeStr=uint8  ZeroCross=off
  Compare To Zero8 : simulink/Logic and Bit Operations/Compare To Zero  relop===  OutDataTypeStr=uint8  ZeroCross=off
  Data Type Conversion1 : DataTypeConversion
  Display5 : Display
  Hold1 : Stateflow chart  TreatAsAtomicUnit=on
  Mux1 : Mux  Inputs=2
  Nan Check : simulink/Model Verification/Check  Static Range  Description=-inf < u < inf  max=inf  max_included=off  min=-inf  min_included=off  enabled=on  stopWhenAssertionFail=off  export=on  icon=graphic
  Sum of Elements : Sum  Inputs=+
  Unit Delay1 : UnitDelay  SampleTime=-1
  reset1 : Constant  Value=0
  Out1 : Outport
  wires:
  In1/1 -> Nan Check/1
  Nan Check/1 -> Display5/1, Compare To Zero6/1
  Compare To Zero6/1 -> Sum of Elements/1
  reset1/1 -> Mux1/2
  Mux1/1 -> Hold1/Trigger
  Hold1/1(error) -> Compare To Zero8/1
  Data Type Conversion1/1 -> Mux1/1
  Unit Delay1/1 -> Data Type Conversion1/1
  Compare To Zero8/1 -> Out1/1
  Sum of Elements/1 -> Unit Delay1/1

== system Copy_of_minimal_rcu_full/Roboter+controller/controller/Joint Impedance/JOINT_IMPEDANCE_CONTROL/Joint Compliance Control/NAN_checks/hold_zero_if_nan_or_inf6 ==
  In1 : Inport
  Compare To Zero6 : simulink/Logic and Bit Operations/Compare To Zero  relop===  OutDataTypeStr=uint8  ZeroCross=off
  Compare To Zero8 : simulink/Logic and Bit Operations/Compare To Zero  relop===  OutDataTypeStr=uint8  ZeroCross=off
  Data Type Conversion1 : DataTypeConversion
  Display5 : Display
  Hold1 : Stateflow chart  TreatAsAtomicUnit=on
  Mux1 : Mux  Inputs=2
  Nan Check : simulink/Model Verification/Check  Static Range  Description=-inf < u < inf  max=inf  max_included=off  min=-inf  min_included=off  enabled=on  stopWhenAssertionFail=off  export=on  icon=graphic
  Sum of Elements : Sum  Inputs=+
  Unit Delay1 : UnitDelay  SampleTime=-1
  reset1 : Constant  Value=0
  Out1 : Outport
  wires:
  Sum of Elements/1 -> Unit Delay1/1
  Compare To Zero8/1 -> Out1/1
  Unit Delay1/1 -> Data Type Conversion1/1
  Data Type Conversion1/1 -> Mux1/1
  Hold1/1(error) -> Compare To Zero8/1
  Mux1/1 -> Hold1/Trigger
  reset1/1 -> Mux1/2
  Compare To Zero6/1 -> Sum of Elements/1
  Nan Check/1 -> Compare To Zero6/1, Display5/1
  In1/1 -> Nan Check/1

== system Copy_of_minimal_rcu_full/Roboter+controller/controller/Joint Impedance/JOINT_IMPEDANCE_CONTROL/Joint Compliance Control/NAN_checks/hold_zero_if_nan_or_inf7 ==
  In1 : Inport
  Compare To Zero6 : simulink/Logic and Bit Operations/Compare To Zero  relop===  OutDataTypeStr=uint8  ZeroCross=off
  Compare To Zero8 : simulink/Logic and Bit Operations/Compare To Zero  relop===  OutDataTypeStr=uint8  ZeroCross=off
  Data Type Conversion1 : DataTypeConversion
  Display5 : Display
  Hold1 : Stateflow chart  TreatAsAtomicUnit=on
  Mux1 : Mux  Inputs=2
  Nan Check : simulink/Model Verification/Check  Static Range  Description=-inf < u < inf  max=inf  max_included=off  min=-inf  min_included=off  enabled=on  stopWhenAssertionFail=off  export=on  icon=graphic
  Sum of Elements : Sum  Inputs=+
  Unit Delay1 : UnitDelay  SampleTime=-1
  reset1 : Constant  Value=0
  Out1 : Outport
  wires:
  In1/1 -> Nan Check/1
  Nan Check/1 -> Display5/1, Compare To Zero6/1
  Compare To Zero6/1 -> Sum of Elements/1
  reset1/1 -> Mux1/2
  Mux1/1 -> Hold1/Trigger
  Hold1/1(error) -> Compare To Zero8/1
  Data Type Conversion1/1 -> Mux1/1
  Unit Delay1/1 -> Data Type Conversion1/1
  Compare To Zero8/1 -> Out1/1
  Sum of Elements/1 -> Unit Delay1/1

== system Copy_of_minimal_rcu_full/Roboter+controller/controller/Joint Impedance/JOINT_IMPEDANCE_CONTROL/Joint Compliance Control/NAN_checks/hold_zero_if_nan_or_inf8 ==
  In1 : Inport
  Compare To Zero6 : simulink/Logic and Bit Operations/Compare To Zero  relop===  OutDataTypeStr=uint8  ZeroCross=off
  Compare To Zero8 : simulink/Logic and Bit Operations/Compare To Zero  relop===  OutDataTypeStr=uint8  ZeroCross=off
  Data Type Conversion1 : DataTypeConversion
  Display5 : Display
  Hold1 : Stateflow chart  TreatAsAtomicUnit=on
  Mux1 : Mux  Inputs=2
  Nan Check : simulink/Model Verification/Check  Static Range  Description=-inf < u < inf  max=inf  max_included=off  min=-inf  min_included=off  enabled=on  stopWhenAssertionFail=off  export=on  icon=graphic
  Sum of Elements : Sum  Inputs=+
  Unit Delay1 : UnitDelay  SampleTime=-1
  reset1 : Constant  Value=0
  Out1 : Outport
  wires:
  Sum of Elements/1 -> Unit Delay1/1
  Compare To Zero8/1 -> Out1/1
  Unit Delay1/1 -> Data Type Conversion1/1
  Data Type Conversion1/1 -> Mux1/1
  Hold1/1(error) -> Compare To Zero8/1
  Mux1/1 -> Hold1/Trigger
  reset1/1 -> Mux1/2
  Compare To Zero6/1 -> Sum of Elements/1
  Nan Check/1 -> Compare To Zero6/1, Display5/1
  In1/1 -> Nan Check/1

== system Copy_of_minimal_rcu_full/Roboter+controller/controller/Joint Impedance/JOINT_IMPEDANCE_CONTROL/Joint Compliance Control/Pragmatic Solution/nan_chk4 ==
  in : Inport
  Add : Sum
  Compare To Zero : simulink/Logic and Bit Operations/Compare To Zero  relop===  OutDataTypeStr=uint8  ZeroCross=off
  Compare To Zero1 : simulink/Logic and Bit Operations/Compare To Zero  relop=>  OutDataTypeStr=uint8  ZeroCross=off
  Constant2 : Constant  Value=sample_time_model
  Discrete Derivative2 : simulink/Discrete/Discrete Derivative  gainval=1.0  ICPrevScaledInput=0.0  InputProcessing=Inherited  OutMin=[]  OutMax=[]  OutDataType=sfix(16)  OutScaling=2^-10  DoSatur=off
  NAN_chk_theta : Display
  Product1 : Product  RndMeth=Zero
  Relational Operator : RelationalOperator  Operator===  OutDataTypeStr=boolean
  Sum of Elements : Sum  Inputs=+
  Switch : Switch  Criteria=u2 > Threshold
  Unit Delay1 : UnitDelay  SampleTime=-1
  in_checked : Outport  PortDimensions=7
  wires:
  Unit Delay1/1 -> Switch/1
  Add/1 -> Unit Delay1/1
  Product1/1 -> Add/2
  Discrete Derivative2/1 -> Product1/1
  Constant2/1 -> Product1/2
  Switch/1 -> Add/1, Discrete Derivative2/1, in_checked/1
  in/1 -> Switch/3, Relational Operator/2, Relational Operator/1
  Relational Operator/1 -> Compare To Zero/1
  Compare To Zero/1 -> Sum of Elements/1
  Sum of Elements/1 -> Compare To Zero1/1
  Compare To Zero1/1 -> Switch/2, NAN_chk_theta/1

== system Copy_of_minimal_rcu_full/Roboter+controller/controller/Cartesian Impedance Control/Subsystem/Cartesian Compliance Control/Cartesian Damping/Cartesian mass matrix/Subsystem1 ==
  note: J*inv(M)*J'
  in_matrix : Inport
  Constant : Constant  Value=MIN_SING_VALUE_M_CART
  inv with hold : MATLAB Function  TreatAsAtomicUnit=on
  not_singular : Outport
  inv_matrix : Outport  Port=2
  inv_matrix_sqrt : Outport  Port=3
  wires:
  Constant/1 -> inv with hold/2(min_singular_value)
  inv with hold/1(not_singular) -> not_singular/1
  in_matrix/1 -> inv with hold/1(in_matrix)
  inv with hold/2(inv_matrix) -> inv_matrix/1
  inv with hold/3(inv_matrix_sqrt) -> inv_matrix_sqrt/1

== system Copy_of_minimal_rcu_full/Roboter+controller/controller/Cartesian Impedance Control/Subsystem/Cartesian Compliance Control/Cartesian Damping/Damping Design via Generalized Eigenvalues/Damping Design via Generalized Eigenvalues QR right ==
  K : Inport
  M : Inport  Port=2
  damp_fac : Inport  Port=3
  2*Damping Fac : Gain  Gain=2
  Double diagonalization : MATLAB Function  TreatAsAtomicUnit=on
  Embedded MATLAB Function : MATLAB Function  TreatAsAtomicUnit=on
  Math Function1 : Math  Operator=sqrt  OutputSignalType=real  SaturateOnIntegerOverflow=on
  Product1 : Product  Inputs=***  Multiplication=Matrix(*)  RndMeth=Zero
  Product2 : Product  Inputs=**  Multiplication=Matrix(*)  RndMeth=Zero
  Product3 : Product  Inputs=**  RndMeth=Zero
  D : Outport
  wires:
  M/1 -> Double diagonalization/2(B), Product2/1
  Math Function1/1 -> 2*Damping Fac/1
  Double diagonalization/1(V) -> Product2/2
  Double diagonalization/3(lambda) -> Math Function1/1
  K/1 -> Double diagonalization/1(A)
  Product1/1 -> D/1
  2*Damping Fac/1 -> Product3/1
  Product3/1 -> Embedded MATLAB Function/1(u)
  damp_fac/1 -> Product3/2
  Product2/1 -> Product1/1
  Embedded MATLAB Function/1(y) -> Product1/2  "C"
  Double diagonalization/2(Vinv) -> Product1/3

== system Copy_of_minimal_rcu_full/Roboter+controller/controller/Cartesian Impedance Control/Subsystem/Cartesian Compliance Control/Iterative Computation of the 'Stiffness' and Gravity Compensation/Iteration for Nolcos Controller/Euler Angle Stiffness ==
  Hsd : Inport
  Fkin : Inport  Port=2
  Jbody : Inport  Port=3
  K : Inport  Port=4
  relaxing : Inport  Port=5
  Enable : EnablePort  StatesWhenEnabling=reset
  Euler Angle Components : Subsystem
  Math Function : Math  Operator=transpose  SaturateOnIntegerOverflow=on
  Matrix Gain : Gain  Gain=-1  SaturateOnIntegerOverflow=on  OutDataTypeStr=Inherit: Same as input  ParamDataTypeStr=Inherit: Same as input
  Product1 : Product  Multiplication=Matrix(*)  RndMeth=Zero
  Product2 : Product  RndMeth=Zero
  Product4 : Product  Multiplication=Matrix(*)  RndMeth=Zero
  Reshape1 : Reshape  OutputDimensionality=Column vector (2-D)
  Reshape2 : Reshape  OutputDimensionality=Column vector (2-D)
  Reshape3 : Reshape
  Reshape4 : Reshape
  tau : Outport
  J : Outport  Port=2
  x : Outport  Port=3
  F : Outport  Port=4
  wires:
  Math Function/1 -> Product4/1
  Euler Angle Components/2(Jx) -> Math Function/1, J/1
  Euler Angle Components/1(x) -> x/1, Reshape1/1
  Fkin/1 -> Euler Angle Components/2(Fkin)
  Hsd/1 -> Euler Angle Components/1(Hsd)
  Jbody/1 -> Euler Angle Components/3(J)
  Product4/1 -> Matrix Gain/1
  Matrix Gain/1 -> Reshape3/1
  K/1 -> Product1/1
  Product1/1 -> Product2/1
  Product2/1 -> Product4/2, Reshape4/1
  relaxing/1 -> Reshape2/1
  Reshape1/1 -> Product1/2
  Reshape2/1 -> Product2/2
  Reshape3/1 -> tau/1
  Reshape4/1 -> F/1

== system Copy_of_minimal_rcu_full/Roboter+controller/controller/Cartesian Impedance Control/Subsystem/Cartesian Compliance Control/Iterative Computation of the 'Stiffness' and Gravity Compensation/Iteration for Nolcos Controller/LBR M Components2 ==
  q : Inport
  load : Inport  Port=2
  tcp_offset : Inport  Port=3
  base_acceleration : Inport  Port=4
  Forward Kinematics LBR-M2 : holgersRobLib/Forward Kinematics LBR-M2
  Jacobian LBR-M : holgersRobLib/Jacobian LBR-M
  S-Function1 : S-Function  FunctionName=lbrmgrav_sfun  EnableBusSupport=off
  Fkin : Outport
  J : Outport  Port=2
  grav : Outport  Port=3
  wires:
  load/1 -> S-Function1/2
  S-Function1/1 -> grav/1
  q/1 -> S-Function1/1, Jacobian LBR-M/1, Forward Kinematics LBR-M2/1
  Jacobian LBR-M/1 -> J/1
  Forward Kinematics LBR-M2/1 -> Fkin/1
  base_acceleration/1 -> S-Function1/3
  tcp_offset/1 -> Forward Kinematics LBR-M2/2, Jacobian LBR-M/2
